simulink model "chap9_4sim"  (Simulink 3.00)
settings: Solver=ode45  StartTime=0.0  StopTime=10  RelTol=1e-3
settings Model: LastModifiedBy=liu

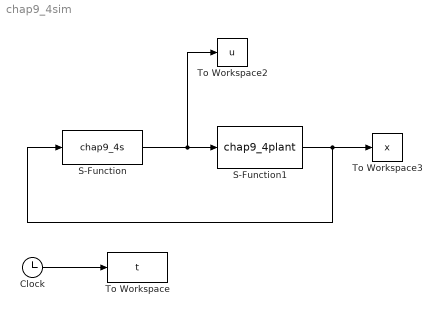
== system chap9_4sim ==
  Clock : Clock
      settings: DisplayTime=off  Decimation=10
  S-Function : S-Function  FunctionName=chap9_4s  PortCounts=[]  SFunctionModules=''
  S-Function1 : S-Function  FunctionName=chap9_4plant  PortCounts=[]  SFunctionModules=''
  To Workspace : ToWorkspace  VariableName=t  SampleTime=-1  SaveFormat=Matrix
  To Workspace2 : ToWorkspace  VariableName=u  SampleTime=-1  SaveFormat=Matrix
  To Workspace3 : ToWorkspace  VariableName=x  SampleTime=-1  SaveFormat=Matrix
  wires:
  S-Function1/1 -> To Workspace3/1, S-Function/1
  S-Function/1 -> S-Function1/1, To Workspace2/1
  Clock/1 -> To Workspace/1
